simulink model "PID_base_simulink"  (R2022b)
settings: Solver=VariableStepAuto  StartTime=0.0  StopTime=10.0  RelTol=1e-3
values from neighbouring files (symbols this model uses):
  A1 = (pi*de^2)/4    (= 0.00502654824574)    [PID_parametros_novos.m]
  A2 = A1-(pi*dh^2)/4    (= 0.00343611696486)    [PID_parametros_novos.m]
  Be = 9000*10^5    (= 900000000)    [PID_parametros_novos.m]
  f = 1500    [PID_parametros_novos.m]
  k = [20 0.02 0.0001]    [genetic_algorithm.m]
  kc1 = 7e-13    [PID_parametros_novos.m]
  kc2 = 1e-12    [PID_parametros_novos.m]
  kq1 = 0.0027459    [PID_parametros_novos.m]
  kq2 = 0.001091    [PID_parametros_novos.m]
  M = Mguias_movida+Me+Mh    (= 91.9784261851)    [PID_parametros_novos.m]
  V1 = Vl1+A1*xe0    (= 0.000442176956151)    [PID_parametros_novos.m]
  V2 = Vl2+A2*(L-xe0)    (= 0.000455461801854)    [PID_parametros_novos.m]
libraries: simulink x1
settings Model: Creator=dsilva  LastModifiedBy=dsilva
settings DataIOCC: ReturnWorkspaceOutputs=off

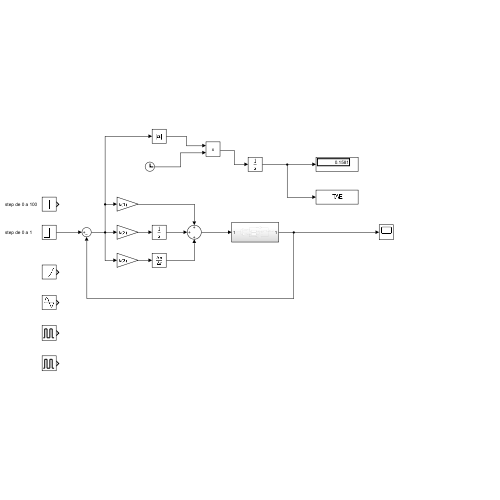
[thumbnail: Simulink's stored preview of the top-level diagram]
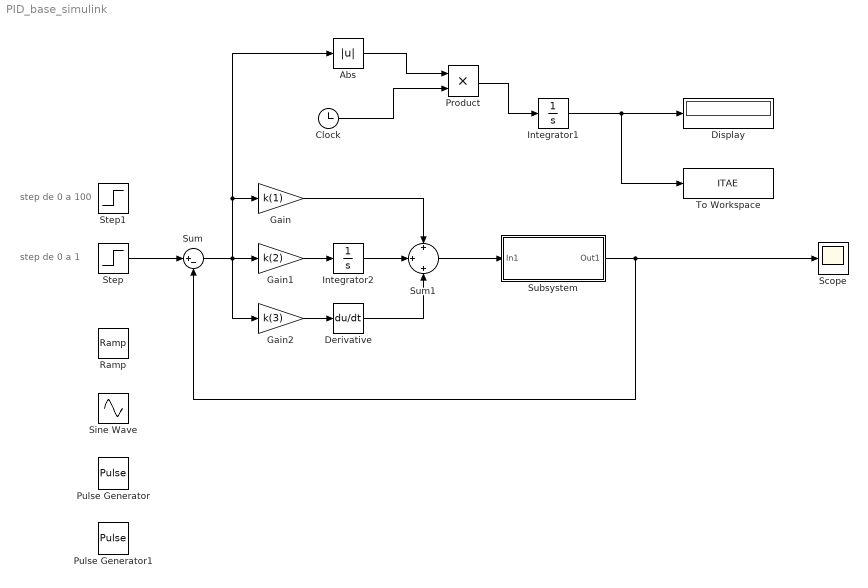
== system PID_base_simulink ==
  note: step de 0 a 1
  note: step de 0 a 100
  Abs : Abs  SaturateOnIntegerOverflow=off
  Clock : Clock
  Derivative : Derivative
  Display : Display
  Gain : Gain  Gain=k(1)
  Gain1 : Gain  Gain=k(2)
  Gain2 : Gain  Gain=k(3)
  Integrator1 : Integrator
  Integrator2 : Integrator
  Product : Product
  Pulse Generator : DiscretePulseGenerator  PulseType=Time based  Period=10  PulseWidth=5
  Pulse Generator1 : DiscretePulseGenerator  PulseType=Time based  Period=10  PulseWidth=20
  Ramp : simulink/Sources/Ramp  slope=1  start=0  InitialOutput=0
  Scope : Scope
  Sine Wave : Sin  Frequency=2  SampleTime=0
  Step : Step  SampleTime=0
  Step1 : Step  SampleTime=0
  Subsystem : Subsystem
  Sum : Sum  Inputs=|+-
  Sum1 : Sum  Inputs=+|+|+
  To Workspace : ToWorkspace  VariableName=ITAE  SampleTime=-1
  wires:
  Gain1/1 -> Integrator2/1
  Sum/1 -> Abs/1, Gain/1, Gain2/1, Gain1/1
  Gain2/1 -> Derivative/1
  Integrator1/1 -> To Workspace/1, Display/1
  Gain/1 -> Sum1/1
  Subsystem/1(Out1) -> Scope/1, Sum/2
  Integrator2/1 -> Sum1/2
  Abs/1 -> Product/1
  Derivative/1 -> Sum1/3
  Sum1/1 -> Subsystem/1(In1)
  Step/1 -> Sum/1
  Clock/1 -> Product/2
  Product/1 -> Integrator1/1

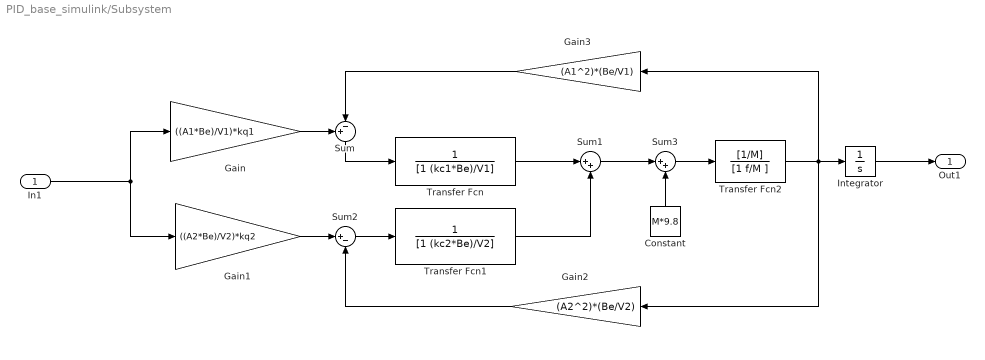
== system PID_base_simulink/Subsystem ==
  In1 : Inport
  Constant : Constant  Value=M*9.8
  Gain : Gain  Gain=((A1*Be)/V1)*kq1
  Gain1 : Gain  Gain=((A2*Be)/V2)*kq2
  Gain2 : Gain  Gain=(A2^2)*(Be/V2)
  Gain3 : Gain  Gain=(A1^2)*(Be/V1)
  Integrator : Integrator
  Sum : Sum  Inputs=+-|
  Sum1 : Sum  Inputs=|++
  Sum2 : Sum  Inputs=|+-
  Sum3 : Sum  Inputs=|++
  Transfer Fcn : TransferFcn  Denominator=[1 (kc1*Be)/V1]
  Transfer Fcn1 : TransferFcn  Denominator=[1 (kc2*Be)/V2]
  Transfer Fcn2 : TransferFcn  Numerator=[1/M]  Denominator=[1 f/M ]
  Out1 : Outport
  wires:
  Sum1/1 -> Sum3/1
  Constant/1 -> Sum3/2
  Gain1/1 -> Sum2/1
  Sum3/1 -> Transfer Fcn2/1
  Transfer Fcn2/1 -> Gain2/1, Gain3/1, Integrator/1
  Gain2/1 -> Sum2/2
  Sum2/1 -> Transfer Fcn1/1
  Transfer Fcn1/1 -> Sum1/2
  Transfer Fcn/1 -> Sum1/1
  In1/1 -> Gain/1, Gain1/1
  Integrator/1 -> Out1/1
  Sum/1 -> Transfer Fcn/1
  Gain3/1 -> Sum/2
  Gain/1 -> Sum/1
